simulink model "RocketLander_version2_2021a_version"  (R2022a)
settings: Solver=VariableStepAuto  StartTime=0.0  StopTime=20  MaxStep=1E-3  RelTol=1e-3
model workspace (MAT data in the model file):
  Gimbal_Angle = 0
  gravity = 1
  mass = 1.2
libraries: simulink x2, aerolibanim x1, shared3dof x1, simulink_extras x1
settings Model: Creator=lukea  LastModifiedBy=laagaard2021
settings ModelReferenceCC: EnableRefExpFcnMdlSchedulingChecks=off
settings RTWCC: Description=Generic Real-Time Target

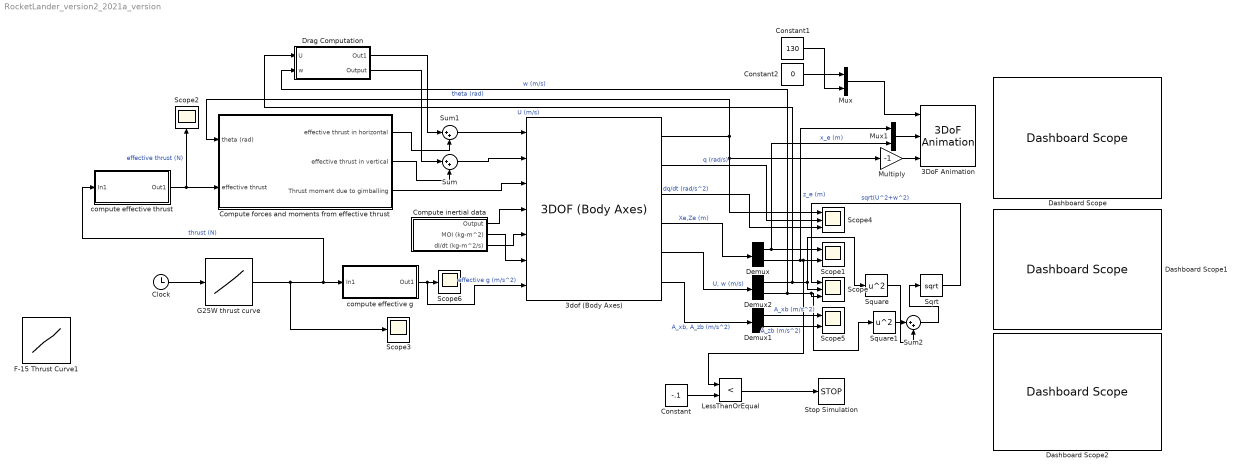
== system RocketLander_version2_2021a_version ==
  3DoF Animation : aerolibanim/3DoF Animation  u1=[-5000 5000 -5000 5000 -5000 5000]  u2=0.05  u3=1  u5=Fly alongside  u6=[50 1000 0]  u7=10  u8=on
      settings: SourceProductBaseCode=AE
  3dof (Body Axes) : shared3dof/3DOF (Body Axes)  units=Metric (MKS)  mtype=Custom Variable  v_ini=0  theta_ini=0  alpha_ini=0  pos_ini=[0 0]  q_ini=0  mass=mass  mass_e=0.5  mass_f=3.0  Iyy=1.5  Iyy_e=0.5  Iyy_f=3.0  g_in=External  g=9.81  vre_flag=off  abi_flag=off  aMode=0  vel_statename=''  theta_statename=''  pos_statename=''  q_statename=''  mass_statename=''
      settings: SourceProductBaseCode=AE,PW,DR,MT,VE
  Clock : Clock
  Compute forces and moments from effective thrust : Subsystem
  Compute inertial data : Subsystem
  Constant : Constant  Value=-.1
  Constant1 : Constant  Value=130
  Constant2 : Constant  Value=0
  Dashboard Scope : DashboardScope
  Dashboard Scope1 : DashboardScope
  Dashboard Scope2 : DashboardScope
  Demux : Demux  Outputs=2
  Demux1 : Demux  Outputs=2
  Demux2 : Demux  Outputs=2
  Drag Computation : Subsystem
  F-15 Thrust Curve1 : Lookup_n-D  NumberOfTableDimensions=1  BreakpointsForDimension1=[0;0.148;0.228;0.294;0.353;0.382;0.419;0.477;0.52;0.593;0.688;0.855;1.037;1.205;1.423;1.452;1.503;1.736;1.955;2.21;2.494;2.763;3.12;3.382;3.404;3.418;3.45]  Table=[0;7.638;12.253;16.391;20.21;22.756;25.26;23.074;20.845;19.093;17.5;16.225;15.427;14.948;14.627;15.741;14.785;14.623;14.303;14.141;13.819;13.338;13.334;13.013;9.352;4.895;0]  ExtrapMethod=Clip  UseLastTableValue=on  InternalRulePriority=Speed  RndMeth=Simplest
  G25W thrust curve : Lookup_n-D  NumberOfTableDimensions=1  BreakpointsForDimension1=[0;0.01;0.029;0.11;0.239;0.496;0.568;0.592;0.749;0.997;1.255;1.498;1.999;2.501;3.006;3.503;3.999;4.371;4.414]  Table=[0;38.046;21.768;30.475;35.775;40.696;42.116;45.429;46.186;45.713;44.198;39.939;31.421;23.093;14.196;7.288;4.07;1.988;0]  ExtrapMethod=Clip  UseLastTableValue=on  InternalRulePriority=Speed  RndMeth=Simplest
  LessThanOrEqual : RelationalOperator  Operator=<  OutDataTypeStr=boolean  RndMeth=Simplest  InputSameDT=off
  Multiply : Gain  Gain=-1
  Mux : Mux  Inputs=2
  Mux1 : Mux  Inputs=2
  Scope : Scope  NumInputPorts=3
  Scope1 : Scope  NumInputPorts=2
  Scope2 : Scope
  Scope3 : Scope
  Scope4 : Scope  NumInputPorts=3
  Scope5 : Scope  NumInputPorts=2
  Scope6 : Scope
  Sqrt : Sqrt
  Square : Math  Operator=square
  Square1 : Math  Operator=square
  Stop Simulation : Stop
  Sum : Sum  Inputs=|++
  Sum1 : Sum  Inputs=|++
  Sum2 : Sum  Inputs=|++
  compute effective g : Subsystem
  compute effective thrust : Subsystem
  wires:
  Clock/1 -> G25W thrust curve/1
  G25W thrust curve/1 -> Scope3/1, compute effective thrust/1(In1), compute effective g/1(In1)  "thrust (N)"
  3dof (Body Axes)/1 -> Compute forces and moments from effective thrust/1(theta (rad)), Multiply/1, Scope4/1  "theta (rad)"
  3dof (Body Axes)/4 -> Demux/1  "Xe,Ze (m)"
  3dof (Body Axes)/6 -> Demux1/1  "A_xb, A_zb (m/s^2)"
  Demux/1 -> Mux1/2, Scope1/1  "x_e (m)"
  3dof (Body Axes)/2 -> Scope4/2  "q (rad/s)"
  3dof (Body Axes)/3 -> Scope4/3  "dq/dt (rad/s^2)"
  3dof (Body Axes)/5 -> Demux2/1  "U, w (m/s)"
  Demux2/1 -> Drag Computation/1(U), Square/1, Scope/2  "U (m/s)"
  Demux2/2 -> Drag Computation/2(w), Square1/1, Scope/3  "w (m/s)"
  Demux1/1 -> Scope5/1  "A_xb (m/s^2)"
  Demux1/2 -> Scope5/2  "A_zb (m/s^2)"
  compute effective g/1(Out1) -> 3dof (Body Axes)/7, Scope6/1  "effective g (m/s^2)"
  compute effective thrust/1(Out1) -> Scope2/1, Compute forces and moments from effective thrust/2(effective thrust)  "effective thrust (N)"
  Compute forces and moments from effective thrust/2(effective thrust in vertical) -> Sum/2
  Compute forces and moments from effective thrust/3(Thrust moment due to gimballing) -> 3dof (Body Axes)/3
  Demux/2 -> Mux1/1, LessThanOrEqual/1, Scope1/2  "z_e (m)"
  Sum/1 -> 3dof (Body Axes)/2
  Sum1/1 -> 3dof (Body Axes)/1
  Compute forces and moments from effective thrust/1(effective thrust in horizontal) -> Sum1/2
  Drag Computation/1(Out1) -> Sum1/1
  Drag Computation/2(Output) -> Sum/1
  LessThanOrEqual/1 -> Stop Simulation/1
  Constant/1 -> LessThanOrEqual/2
  Compute inertial data/1(Output) -> 3dof (Body Axes)/4
  Compute inertial data/2(MOI (kg-m^2)) -> 3dof (Body Axes)/6
  Compute inertial data/3(dI/dt (kg-m^2/s)) -> 3dof (Body Axes)/5
  Square/1 -> Sum2/2
  Sum2/1 -> Sqrt/1
  Square1/1 -> Sum2/1
  Sqrt/1 -> Scope/1  "sqrt(U^2+w^2)"
  Mux/1 -> 3DoF Animation/1
  Constant2/1 -> Mux/1
  Constant1/1 -> Mux/2
  Mux1/1 -> 3DoF Animation/2
  Multiply/1 -> 3DoF Animation/3

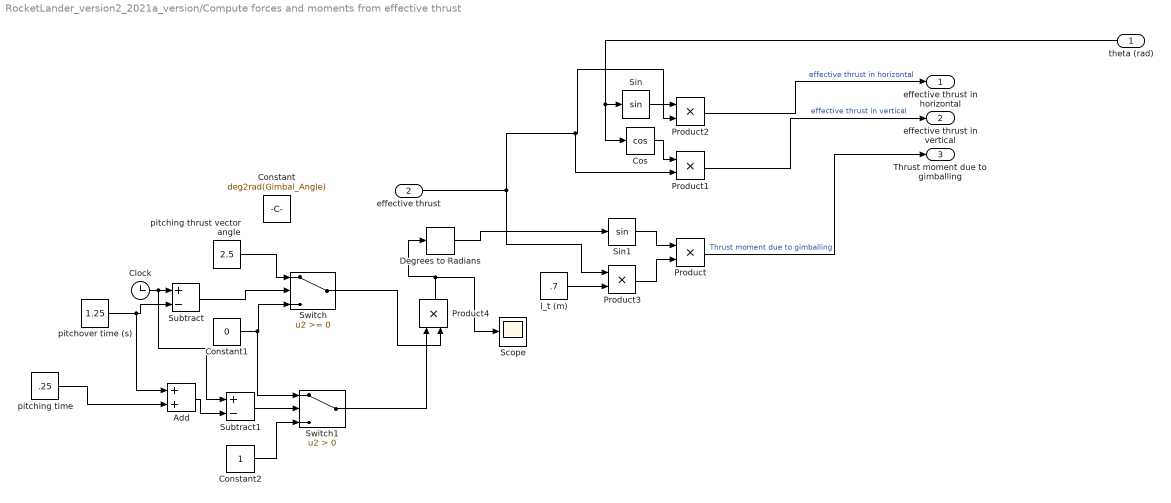
== system RocketLander_version2_2021a_version/Compute forces and moments from effective thrust ==
  theta (rad) : Inport
  effective thrust : Inport  Port=2
  Add : Sum
  Clock : Clock
  Constant : Constant  Value=deg2rad(Gimbal_Angle)
  Constant1 : Constant  Value=0
  Constant2 : Constant
  Cos : Trigonometry  Operator=cos
  Degrees to Radians : simulink_extras/Transformations/Degrees to Radians
  Product{,1..4} (5 alike) : Product
  Scope : Scope
  Sin : Trigonometry
  Sin1 : Trigonometry
  Subtract : Sum  Inputs=+-
  Subtract1 : Sum  Inputs=+-
  Switch : Switch  SaturateOnIntegerOverflow=off  InputSameDT=off
  Switch1 : Switch  Criteria=u2 > Threshold  SaturateOnIntegerOverflow=off  InputSameDT=off
  l_t (m) : Constant  Value=.7
  pitching thrust vector angle : Constant  Value=2.5
  pitching time : Constant  Value=.25
  pitchover time (s) : Constant  Value=1.25
  effective thrust in horizontal : Outport
  effective thrust in vertical : Outport  Port=2
  Thrust moment due to gimballing : Outport  Port=3
  wires:
  Cos/1 -> Product1/1
  effective thrust/1 -> Product1/2, Product2/2, Product3/1
  theta (rad)/1 -> Sin/1, Cos/1
  Sin/1 -> Product2/1
  Sin1/1 -> Product/1
  Product/1 -> Thrust moment due to gimballing/1  "Thrust moment due to gimballing"
  Product3/1 -> Product/2
  l_t (m)/1 -> Product3/2
  Product1/1 -> effective thrust in vertical/1  "effective thrust in vertical"
  Product2/1 -> effective thrust in horizontal/1  "effective thrust in horizontal"
  Clock/1 -> Subtract1/1, Subtract/1
  pitchover time (s)/1 -> Add/1, Subtract/2
  Subtract/1 -> Switch/2
  pitching thrust vector angle/1 -> Switch/1
  Constant1/1 -> Switch1/1, Switch/3
  pitching time/1 -> Add/2
  Add/1 -> Subtract1/2
  Subtract1/1 -> Switch1/2
  Switch1/1 -> Product4/1
  Constant2/1 -> Switch1/3
  Switch/1 -> Product4/2
  Product4/1 -> Degrees to Radians/1, Scope/1
  Degrees to Radians/1 -> Sin1/1

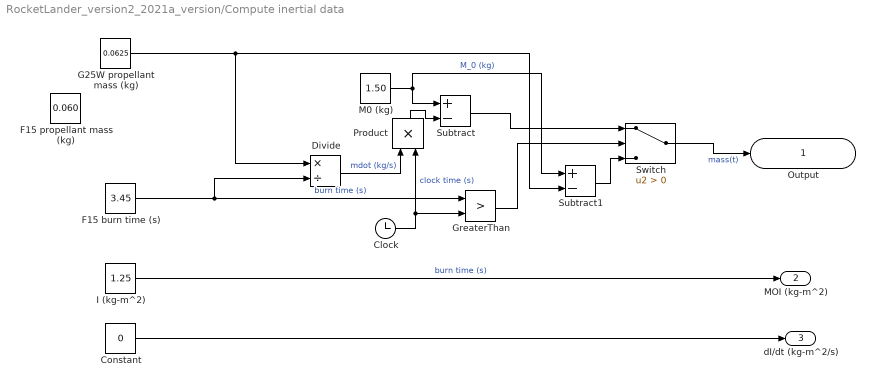
== system RocketLander_version2_2021a_version/Compute inertial data ==
  Clock : Clock
  Constant : Constant  Value=0
  Divide : Product  Inputs=*/
  F15 burn time (s) : Constant  Value=3.45
  F15 propellant mass (kg) : Constant  Value=0.060
  G25W propellant mass (kg) : Constant  Value=0.0625
  GreaterThan : RelationalOperator  Operator=>  OutDataTypeStr=boolean  RndMeth=Simplest  InputSameDT=off
  I (kg-m^2) : Constant  Value=1.25
  M0 (kg) : Constant  Value=1.50
  Product : Product
  Subtract : Sum  Inputs=+-
  Subtract1 : Sum  Inputs=+-
  Switch : Switch  Criteria=u2 > Threshold  SaturateOnIntegerOverflow=off  InputSameDT=off
  Output : Outport
  MOI (kg-m^2) : Outport  Port=2
  dI/dt (kg-m^2/s) : Outport  Port=3
  wires:
  Switch/1 -> Output/1  "mass(t)"
  Clock/1 -> GreaterThan/2, Product/2  "clock time (s)"
  F15 burn time (s)/1 -> Divide/2, GreaterThan/1  "burn time (s)"
  GreaterThan/1 -> Switch/2
  Subtract/1 -> Switch/1
  M0 (kg)/1 -> Subtract1/1, Subtract/1  "M_0 (kg)"
  Divide/1 -> Product/1  "mdot (kg/s)"
  Product/1 -> Subtract/2
  Subtract1/1 -> Switch/3
  I (kg-m^2)/1 -> MOI (kg-m^2)/1  "burn time (s)"
  Constant/1 -> dI/dt (kg-m^2/s)/1
  G25W propellant mass (kg)/1 -> Divide/1, Subtract1/2

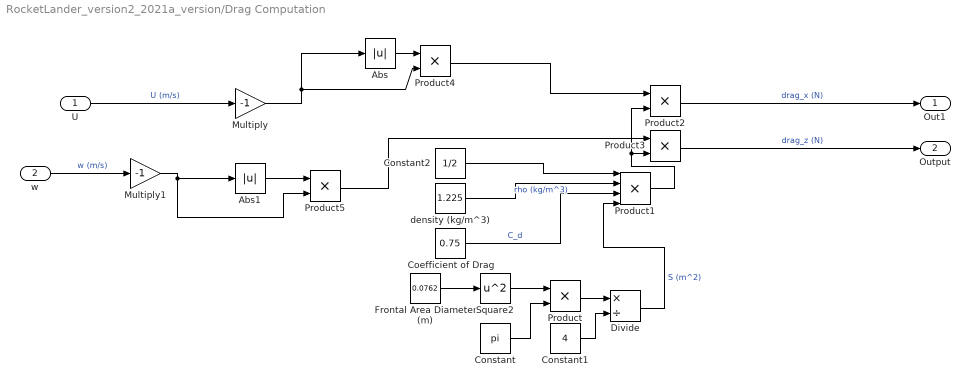
== system RocketLander_version2_2021a_version/Drag Computation ==
  U : Inport
  w : Inport  Port=2
  Abs : Abs  SaturateOnIntegerOverflow=off
  Abs1 : Abs  SaturateOnIntegerOverflow=off
  Coefficient of Drag : Constant  Value=0.75
  Constant : Constant  Value=pi
  Constant1 : Constant  Value=4
  Constant2 : Constant  Value=1/2
  Divide : Product  Inputs=*/
  Frontal Area Diameter (m) : Constant  Value=0.0762
  Multiply : Gain  Gain=-1
  Multiply1 : Gain  Gain=-1
  Product{,2..5} (5 alike) : Product
  Product1 : Product  Inputs=4
  Square2 : Math  Operator=square
  density (kg/m^3) : Constant  Value=1.225
  Out1 : Outport
  Output : Outport  Port=2
  wires:
  Frontal Area Diameter (m)/1 -> Square2/1
  Square2/1 -> Product/1
  Constant/1 -> Product/2
  Product/1 -> Divide/1
  Constant1/1 -> Divide/2
  Divide/1 -> Product1/4  "S (m^2)"
  Coefficient of Drag/1 -> Product1/3  "C_d"
  density (kg/m^3)/1 -> Product1/2  "rho (kg/m^3)"
  Product1/1 -> Product2/2, Product3/2
  Product2/1 -> Out1/1  "drag_x (N)"
  Product3/1 -> Output/1  "drag_z (N)"
  Constant2/1 -> Product1/1
  Product4/1 -> Product2/1
  U/1 -> Multiply/1  "U (m/s)"
  Abs/1 -> Product4/1
  Product5/1 -> Product3/1
  w/1 -> Multiply1/1  "w (m/s)"
  Abs1/1 -> Product5/1
  Multiply/1 -> Abs/1, Product4/2
  Multiply1/1 -> Product5/2, Abs1/1

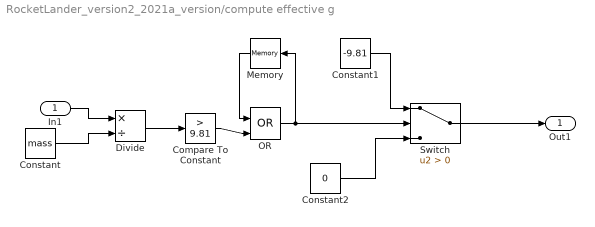
== system RocketLander_version2_2021a_version/compute effective g ==
  In1 : Inport
  Compare To Constant : simulink/Logic and Bit Operations/Compare To Constant  relop=>  const=9.81  OutDataTypeStr=boolean
  Constant : Constant  Value=mass
  Constant1 : Constant  Value=-9.81
  Constant2 : Constant  Value=0
  Divide : Product  Inputs=*/
  Memory : Memory
  OR : Logic  Operator=OR  IconShape=distinctive  AllPortsSameDT=off  OutDataTypeStr=boolean
  Switch : Switch  Criteria=u2 > Threshold  SaturateOnIntegerOverflow=off  InputSameDT=off
  Out1 : Outport
  wires:
  In1/1 -> Divide/1
  Constant/1 -> Divide/2
  Divide/1 -> Compare To Constant/1
  Compare To Constant/1 -> OR/2
  OR/1 -> Switch/2, Memory/1
  Memory/1 -> OR/1
  Constant1/1 -> Switch/1
  Constant2/1 -> Switch/3
  Switch/1 -> Out1/1

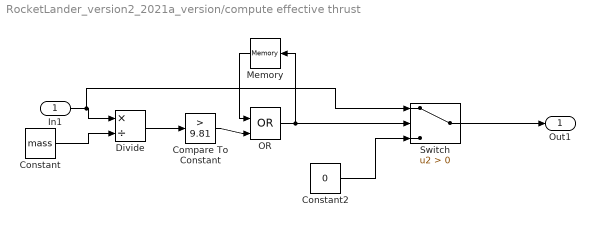
== system RocketLander_version2_2021a_version/compute effective thrust ==
  In1 : Inport
  Compare To Constant : simulink/Logic and Bit Operations/Compare To Constant  relop=>  const=9.81  OutDataTypeStr=boolean
  Constant : Constant  Value=mass
  Constant2 : Constant  Value=0
  Divide : Product  Inputs=*/
  Memory : Memory
  OR : Logic  Operator=OR  IconShape=distinctive  AllPortsSameDT=off  OutDataTypeStr=boolean
  Switch : Switch  Criteria=u2 > Threshold  SaturateOnIntegerOverflow=off  InputSameDT=off
  Out1 : Outport
  wires:
  Constant/1 -> Divide/2
  Divide/1 -> Compare To Constant/1
  Compare To Constant/1 -> OR/2
  OR/1 -> Switch/2, Memory/1
  Memory/1 -> OR/1
  In1/1 -> Switch/1, Divide/1
  Constant2/1 -> Switch/3
  Switch/1 -> Out1/1
